simulink library "Dampers_Axle3_Independent"  (R2026a)
settings: Solver=VariableStepAuto
libraries: Damper_Element x6, fl_lib x6
Description:
  | Component of Simscape Vehicle Templates Library
  | 
  | Copyright 2018-2026 The MathWorks, Inc.
settings Model: Creator=smiller  LastModifiedBy=smiller

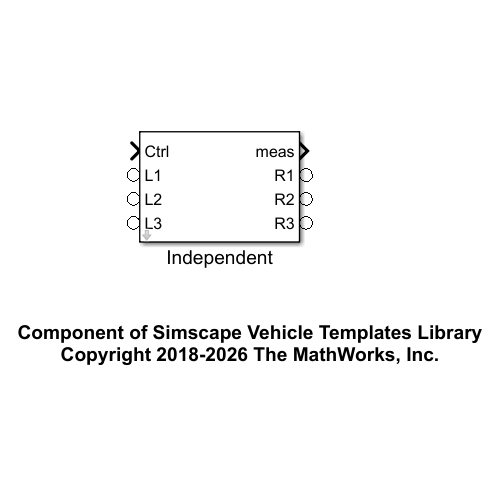
[thumbnail: Simulink's stored preview of the top-level diagram]
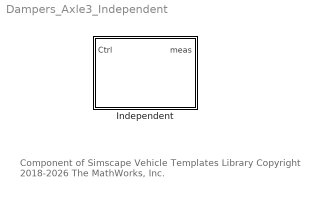
== system Dampers_Axle3_Independent ==
  note: Component of Simscape Vehicle Templates Library
      | Copyright 2018-2026 The MathWorks, Inc.
  Independent : Subsystem  VariantControl=Independent  mask(Independent Dampers){}
      mask help: Models independent left and right dampers.

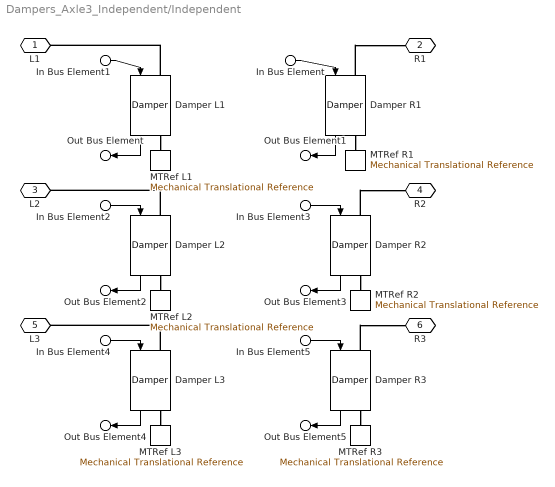
== system Dampers_Axle3_Independent/Independent ==
  In Bus Element1 : Inport  PortName=Ctrl  Element=L1
  In Bus Element : Inport  PortName=Ctrl  Element=R1
  In Bus Element2 : Inport  PortName=Ctrl  Element=L2
  In Bus Element3 : Inport  PortName=Ctrl  Element=R2
  In Bus Element4 : Inport  PortName=Ctrl  Element=L3
  In Bus Element5 : Inport  PortName=Ctrl  Element=R3
  Damper L1 : Damper_Element/Damper  VariantControl=Variant1  LabelModeActiveChoice=Linear  Damper=Damper.Axle1  VariantLabel=Damper.Axle1.class.Value
      settings: AttributesFormatString=%<ActiveVariant>
  Damper L2 : Damper_Element/Damper  VariantControl=Variant1  LabelModeActiveChoice=Linear  Damper=Damper.Axle2  VariantLabel=Damper.Axle2.class.Value
      settings: AttributesFormatString=%<ActiveVariant>
  Damper L3 : Damper_Element/Damper  VariantControl=Variant1  LabelModeActiveChoice=Linear  Damper=Damper.Axle3  VariantLabel=Damper.Axle3.class.Value
      settings: AttributesFormatString=%<ActiveVariant>
  Damper R1 : Damper_Element/Damper  VariantControl=Variant1  LabelModeActiveChoice=Linear  Damper=Damper.Axle1  VariantLabel=Damper.Axle1.class.Value
      settings: AttributesFormatString=%<ActiveVariant>
  Damper R2 : Damper_Element/Damper  VariantControl=Variant1  LabelModeActiveChoice=Linear  Damper=Damper.Axle2  VariantLabel=Damper.Axle2.class.Value
      settings: AttributesFormatString=%<ActiveVariant>
  Damper R3 : Damper_Element/Damper  VariantControl=Variant1  LabelModeActiveChoice=Linear  Damper=Damper.Axle3  VariantLabel=Damper.Axle3.class.Value
      settings: AttributesFormatString=%<ActiveVariant>
  MTRef L1 : fl_lib/Mechanical/Translational Elements/Mechanical Translational Reference
  MTRef L2 : fl_lib/Mechanical/Translational Elements/Mechanical Translational Reference
  MTRef L3 : fl_lib/Mechanical/Translational Elements/Mechanical Translational Reference
  MTRef R1 : fl_lib/Mechanical/Translational Elements/Mechanical Translational Reference
  MTRef R2 : fl_lib/Mechanical/Translational Elements/Mechanical Translational Reference
  MTRef R3 : fl_lib/Mechanical/Translational Elements/Mechanical Translational Reference
  L1 : PMIOPort  Side=Left
  R1 : PMIOPort  Port=2  Side=Right
  L2 : PMIOPort  Port=3  Side=Left
  R2 : PMIOPort  Port=4  Side=Right
  L3 : PMIOPort  Port=5  Side=Left
  R3 : PMIOPort  Port=6  Side=Right
  Out Bus Element : Outport  VectorParamsAs1DForOutWhenUnconnected=off  PortName=meas  Element=L1
  Out Bus Element1 : Outport  VectorParamsAs1DForOutWhenUnconnected=off  PortName=meas  Element=R1
  Out Bus Element2 : Outport  VectorParamsAs1DForOutWhenUnconnected=off  PortName=meas  Element=L2
  Out Bus Element3 : Outport  VectorParamsAs1DForOutWhenUnconnected=off  PortName=meas  Element=R2
  Out Bus Element4 : Outport  VectorParamsAs1DForOutWhenUnconnected=off  PortName=meas  Element=L3
  Out Bus Element5 : Outport  VectorParamsAs1DForOutWhenUnconnected=off  PortName=meas  Element=R3
  wires:
  Damper R2/1 -> Out Bus Element3/1
  Damper L2/1 -> Out Bus Element2/1
  In Bus Element2/1 -> Damper L2/1
  In Bus Element3/1 -> Damper R2/1
  Damper R1/1 -> Out Bus Element1/1
  Damper L1/1 -> Out Bus Element/1
  In Bus Element1/1 -> Damper L1/1
  In Bus Element/1 -> Damper R1/1
  In Bus Element5/1 -> Damper R3/1
  In Bus Element4/1 -> Damper L3/1
  Damper L3/1 -> Out Bus Element4/1
  Damper R3/1 -> Out Bus Element5/1
  connections:
  Damper L1/RConn1 -- MTRef L1/LConn1
  Damper L1/LConn1 -- L1/RConn1
  Damper L2/RConn1 -- MTRef L2/LConn1
  Damper L2/LConn1 -- L2/RConn1
  Damper R2/RConn1 -- MTRef R2/LConn1
  Damper R2/LConn1 -- R2/RConn1
  Damper R1/RConn1 -- MTRef R1/LConn1
  Damper R1/LConn1 -- R1/RConn1
  Damper R3/RConn1 -- MTRef R3/LConn1
  Damper L3/LConn1 -- L3/RConn1
  Damper L3/RConn1 -- MTRef L3/LConn1
  Damper R3/LConn1 -- R3/RConn1
